simulink model "Problem_16_5"  (Simulink 7.5)
settings: Solver=ode45  StartTime=0.0  StopTime=1000  RelTol=1e-3
settings Model: Creator=Holly  LastModifiedBy=Holly

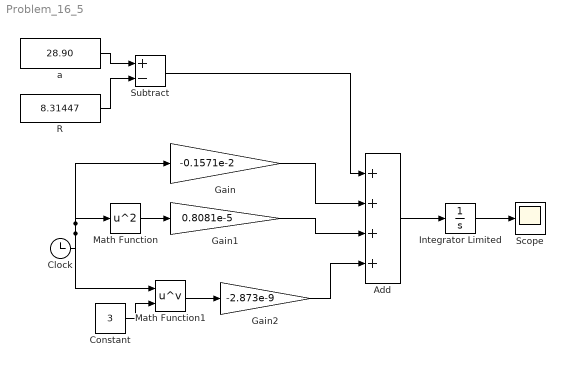
== system Problem_16_5 ==
  Add : Sum  Inputs=++++  OutDataType=fixdt(1, 16)  OutScaling=2^-10
  Clock : Clock
      settings: Decimation=10
  Constant : Constant  Value=3  OutDataType=fixdt(1, 16)  OutScaling=2^0
  Gain : Gain  Gain=-0.1571e-2  ParameterDataType=fixdt(1, 16)  ParameterScaling=2^0  OutDataType=fixdt(1, 16)  OutScaling=2^0
  Gain1 : Gain  Gain=0.8081e-5  ParameterDataType=fixdt(1, 16)  ParameterScaling=2^0  OutDataType=fixdt(1, 16)  OutScaling=2^0
  Gain2 : Gain  Gain=-2.873e-9  ParameterDataType=fixdt(1, 16)  ParameterScaling=2^0  OutDataType=fixdt(1, 16)  OutScaling=2^0
  Integrator Limited : Integrator  UpperSaturationLimit=1  LowerSaturationLimit=0
  Math Function : Math  Operator=square  OutDataType=fixdt(1, 16)  OutScaling=2^0  SaturateOnIntegerOverflow=on
  Math Function1 : Math  Operator=pow  OutDataType=fixdt(1, 16)  OutScaling=2^0  SaturateOnIntegerOverflow=on
  R : Constant  Value=8.31447  OutDataType=fixdt(1, 16)  OutScaling=2^0
  Scope : Scope
  Subtract : Sum  Inputs=+-  OutDataType=fixdt(1, 16)  OutScaling=2^-10
  a : Constant  Value=28.90  OutDataType=fixdt(1, 16)  OutScaling=2^0
  wires:
  a/1 -> Subtract/1
  R/1 -> Subtract/2
  Clock/1 -> Gain/1, Math Function/1, Math Function1/1
  Math Function/1 -> Gain1/1
  Constant/1 -> Math Function1/2
  Math Function1/1 -> Gain2/1
  Subtract/1 -> Add/1
  Gain/1 -> Add/2
  Gain1/1 -> Add/3
  Gain2/1 -> Add/4
  Add/1 -> Integrator Limited/1
  Integrator Limited/1 -> Scope/1
